simulink model "test_simulation"  (R2019b)
settings: Solver=VariableStepAuto  StartTime=0.0  StopTime=10.0  RelTol=1e-3
values from neighbouring files (symbols this model uses):
  Cv = 16.5    [Parameters_Init.m]
  g = 9.81    [AngleToPosition.m]    (also in Parameters_Init.m; plateToBallLinear.m)
  K = 11    [Parameters_Init.m]
  m = 0    [AngleToPosition.m]    (also in Parameters_Init.m = 0.345333333333)
libraries: powerlib_meascontrol x2
settings Model: Creator=123  LastModifiedBy=123

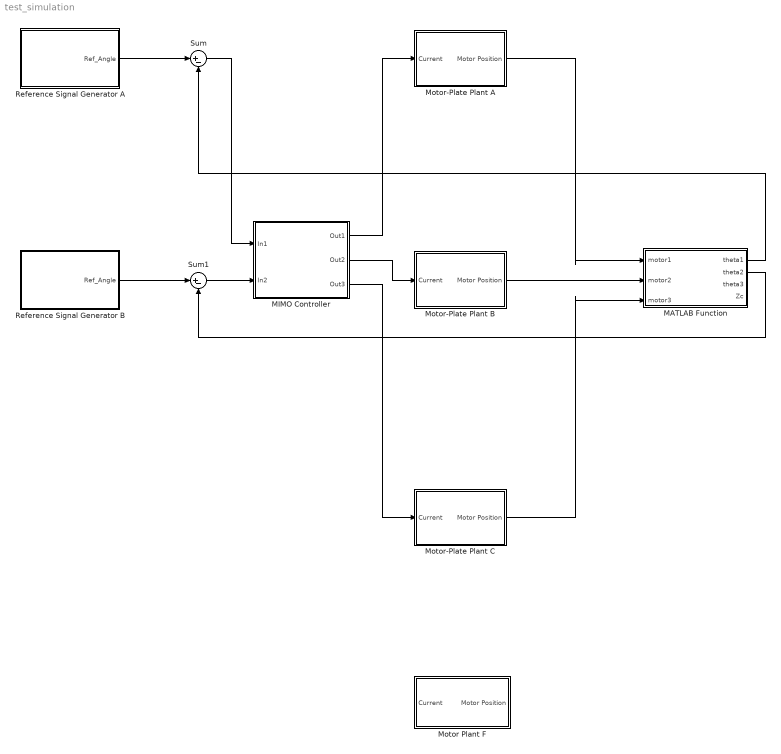
== system test_simulation ==
  MATLAB Function : MATLAB Function  TreatAsAtomicUnit=on
  MIMO Controller : Subsystem
  Motor Plant F : Subsystem
  Motor-Plate Plant A : Subsystem
  Motor-Plate Plant B : Subsystem
  Motor-Plate Plant C : Subsystem
  Reference Signal Generator A : Subsystem
  Reference Signal Generator B : Subsystem
  Sum : Sum  Inputs=|+-
  Sum1 : Sum  Inputs=|+-
  wires:
  MIMO Controller/1(Out1) -> Motor-Plate Plant A/1(Current)
  MIMO Controller/2(Out2) -> Motor-Plate Plant B/1(Current)
  Motor-Plate Plant B/1(Motor Position) -> MATLAB Function/2(motor2)
  Motor-Plate Plant A/1(Motor Position) -> MATLAB Function/1(motor1)
  Motor-Plate Plant C/1(Motor Position) -> MATLAB Function/3(motor3)
  MATLAB Function/1(theta1) -> Sum/2
  Reference Signal Generator A/1(Ref_Angle) -> Sum/1
  Sum/1 -> MIMO Controller/1(In1)
  Reference Signal Generator B/1(Ref_Angle) -> Sum1/1
  Sum1/1 -> MIMO Controller/2(In2)
  MATLAB Function/2(theta2) -> Sum1/2
  MIMO Controller/3(Out3) -> Motor-Plate Plant C/1(Current)

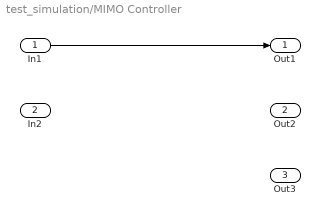
== system test_simulation/MIMO Controller ==
  In1 : Inport
  In2 : Inport  Port=2
  Out1 : Outport
  Out2 : Outport  Port=2
  Out3 : Outport  Port=3
  wires:
  In1/1 -> Out1/1

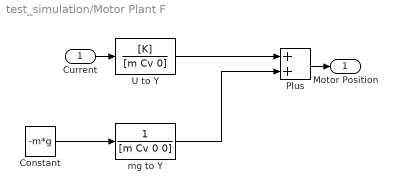
== system test_simulation/Motor Plant F ==
  Current : Inport
  Constant : Constant  Value=-m*g
  Plus : Sum
  U to Y : TransferFcn  Numerator=[K]  Denominator=[m Cv 0]
  mg to Y : TransferFcn  Denominator=[m Cv 0 0]
  Motor Position : Outport
  wires:
  Constant/1 -> mg to Y/1
  Current/1 -> U to Y/1
  Plus/1 -> Motor Position/1
  U to Y/1 -> Plus/1
  mg to Y/1 -> Plus/2

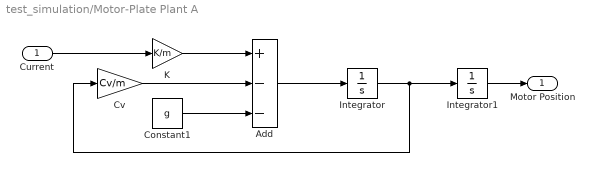
== system test_simulation/Motor-Plate Plant A ==
  Current : Inport
  Add : Sum  Inputs=+--
  Constant1 : Constant  Value=g
  Cv : Gain  Gain=Cv/m
  Integrator : Integrator
  Integrator1 : Integrator
  K : Gain  Gain=K/m
  Motor Position : Outport
  wires:
  Cv/1 -> Add/2
  Add/1 -> Integrator/1
  K/1 -> Add/1
  Integrator1/1 -> Motor Position/1
  Integrator/1 -> Cv/1, Integrator1/1
  Constant1/1 -> Add/3
  Current/1 -> K/1

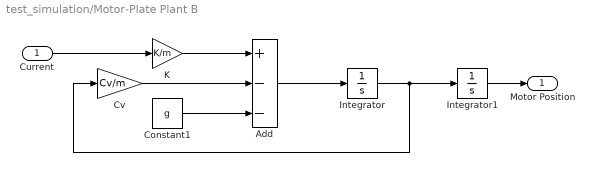
== system test_simulation/Motor-Plate Plant B ==
  Current : Inport
  Add : Sum  Inputs=+--
  Constant1 : Constant  Value=g
  Cv : Gain  Gain=Cv/m
  Integrator : Integrator
  Integrator1 : Integrator
  K : Gain  Gain=K/m
  Motor Position : Outport
  wires:
  Cv/1 -> Add/2
  Add/1 -> Integrator/1
  K/1 -> Add/1
  Integrator1/1 -> Motor Position/1
  Integrator/1 -> Cv/1, Integrator1/1
  Constant1/1 -> Add/3
  Current/1 -> K/1

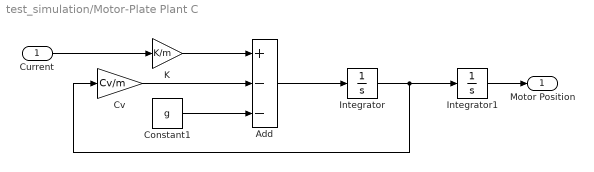
== system test_simulation/Motor-Plate Plant C ==
  Current : Inport
  Add : Sum  Inputs=+--
  Constant1 : Constant  Value=g
  Cv : Gain  Gain=Cv/m
  Integrator : Integrator
  Integrator1 : Integrator
  K : Gain  Gain=K/m
  Motor Position : Outport
  wires:
  Cv/1 -> Add/2
  Add/1 -> Integrator/1
  K/1 -> Add/1
  Integrator1/1 -> Motor Position/1
  Integrator/1 -> Cv/1, Integrator1/1
  Constant1/1 -> Add/3
  Current/1 -> K/1

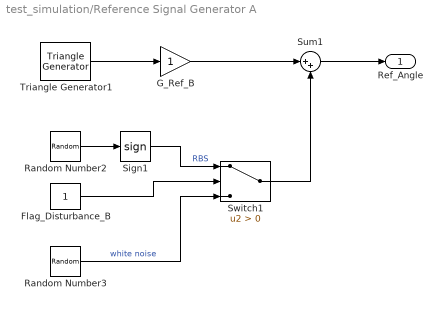
== system test_simulation/Reference Signal Generator A ==
  Flag_Disturbance_B : Constant
  G_Ref_B : Gain
  Random Number2 : RandomNumber  SampleTime=0.001
  Random Number3 : RandomNumber  SampleTime=0.001
  Sign1 : Signum
  Sum1 : Sum  Inputs=|++
  Switch1 : Switch  Criteria=u2 > Threshold
  Triangle Generator1 : powerlib_meascontrol/Pulse & Signal Generators/Triangle Generator  Freq=0.5  Phase=90  Ts=0
      settings: SourceProductName=Simscape Electrical
  Ref_Angle : Outport
  wires:
  Random Number3/1 -> Switch1/3  "white noise"
  Sign1/1 -> Switch1/1  "RBS"
  Random Number2/1 -> Sign1/1
  Switch1/1 -> Sum1/2
  Triangle Generator1/1 -> G_Ref_B/1
  Flag_Disturbance_B/1 -> Switch1/2
  G_Ref_B/1 -> Sum1/1
  Sum1/1 -> Ref_Angle/1

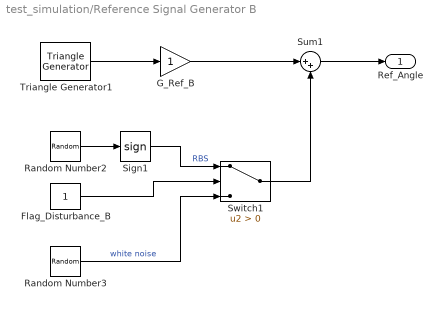
== system test_simulation/Reference Signal Generator B ==
  Flag_Disturbance_B : Constant
  G_Ref_B : Gain
  Random Number2 : RandomNumber  SampleTime=0.001
  Random Number3 : RandomNumber  SampleTime=0.001
  Sign1 : Signum
  Sum1 : Sum  Inputs=|++
  Switch1 : Switch  Criteria=u2 > Threshold
  Triangle Generator1 : powerlib_meascontrol/Pulse & Signal Generators/Triangle Generator  Freq=0.5  Phase=90  Ts=0
      settings: SourceProductName=Simscape Electrical
  Ref_Angle : Outport
  wires:
  Random Number3/1 -> Switch1/3  "white noise"
  Sign1/1 -> Switch1/1  "RBS"
  Random Number2/1 -> Sign1/1
  Switch1/1 -> Sum1/2
  Triangle Generator1/1 -> G_Ref_B/1
  Flag_Disturbance_B/1 -> Switch1/2
  G_Ref_B/1 -> Sum1/1
  Sum1/1 -> Ref_Angle/1

== matlab function test_simulation/MATLAB Function ==
  data: motor1 input; theta1 output; motor2 input; motor3 input; theta2 output; theta3 output; Zc output
function [theta1,theta2,theta3,Zc] = motorsToAngles(motor1, motor2, motor3)

%% Define parameters
r = 0.17;
r0B1 = [r; 0; 0];      
r0B2 = [-0.5*r; (sqrt(3)/2)*r; 0];
r0B3 = [-0.5*r; -(sqrt(3)/2)*r; 0];
r0B = [r0B1 r0B2 r0B3];
%r1C1 = r0B1; r1C2 = r0B2; r1C3 = r0B3;
r1C = r0B;

%% Find Zc
Zc = 1/3*(motor1+motor2+motor3);
r0Oc = [0;0;Zc];

%% Assemble matrices
rBC = [0 0 0; 0 0 0; motor1 motor2 motor3];
r0OC = [r0Oc r0Oc r0Oc];

%% Find A10 (Using \ operator to solve a system of linear equation since the matrix r1C is singular)
A10 = (r1C')\((rBC+r0B-r0OC)');

%% Find angles
theta2 = asin(-A10(1,3));
theta1 = asin(1/cos(theta2)*A10(2,3));
theta3 = asin(1/cos(theta2)*A10(1,2));
end
